simulink model "hexacopter"  (R2014a)
settings: Solver=ode45  StartTime=0.0  StopTime=100  MaxStep=0.5  RelTol=1e-3
undefined symbols (not defined in the file): g, Gt, K, M, m, MU0, obstacle, Qt, RangeFinderParam, Rt, SIGMA0, TP, vt
libraries: commnoisgen2 x2
settings Model: Creator=nirvana1289  LastModifiedBy=nirvana1289
settings DebuggingCC: UnderspecifiedInitializationDetection=Classic  StateNameClashWarn=warning

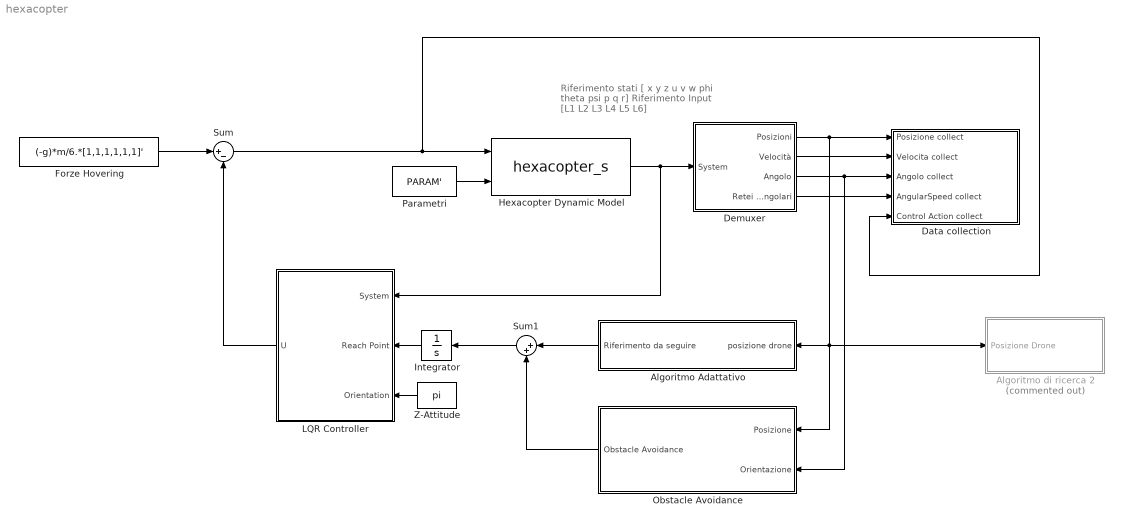
== system hexacopter ==
  note: Riferimento stati
      | [ x y z u v w phi theta psi p q r]
      | Riferimento Input
      | [L1 L2 L3 L4 L5 L6]
  Algoritmo Adattativo : Subsystem
  Algoritmo di ricerca 2 : Subsystem  Commented=on
  Data collection : Subsystem
  Demuxer : Subsystem
  Forze Hovering : Constant  Value=(-g)*m/6.*[1,1,1,1,1,1]'
  Hexacopter Dynamic Model : S-Function  InitFcn=try, set_param(gcb,'FunctionName','hexacopter_s'), end  FunctionName=hexacopter_s  SFunctionModules=hexacopter_s_wrapper  EnableBusSupport=off  mask(S-Function Builder){}
      mask help: Simulink:masks:SFunctionBuilder_MD
      mask init:
      | val = [[.9  0.75 0.75 1 1 .9 .9 1]',[1 1 0.75 0.75 .9 .9 1 .9]'];try , sys = get_param(gcb,'SfunBuilderFcnName');if isempty(sys), sys = get_param(gcb,'FunctionName'); end,catch, sys = get_param(gcb,'FunctionName'); end
      settings: CopyFcn=set_param(gcbh,'LinkStatus','none')  PreSaveFcn=try, set_param(gcb,'FunctionName','hexacopter_s'), end  OpenFcn=sfunctionwizard(gcbh)
      mask Display:
      | plot(val(:,1),val(:,2))
      | disp(sys)
      | port_label('input',1,'u')
      | port_label('input',2,'p')
      | port_label('output',1,'y')
  Integrator : Integrator  InitialCondition=RP'
  LQR Controller : Subsystem
  Obstacle Avoidance : Subsystem
  Parametri : Constant  Value=PARAM'
  Sum : Sum  Inputs=|+-
  Sum1 : Sum  Inputs=|++
  Z-Attitude : Constant  Value=pi
  wires:
  Sum/1 -> Hexacopter Dynamic Model/1, Data collection/5(Control Action collect)
  Forze Hovering/1 -> Sum/1
  Demuxer/3(Angolo) -> Obstacle Avoidance/2(Orientazione), Data collection/3(Angolo collect)
  Demuxer/4(Retei angolari) -> Data collection/4(AngularSpeed collect)
  Demuxer/2(Velocità) -> Data collection/2(Velocita collect)
  Demuxer/1(Posizioni) -> Obstacle Avoidance/1(Posizione), Algoritmo Adattativo/1(posizione drone), Algoritmo di ricerca 2/1(Posizione Drone), Data collection/1(Posizione collect)
  Parametri/1 -> Hexacopter Dynamic Model/2
  LQR Controller/1(U) -> Sum/2
  Z-Attitude/1 -> LQR Controller/3(Orientation)
  Hexacopter Dynamic Model/1 -> LQR Controller/1(System), Demuxer/1(System)
  Integrator/1 -> LQR Controller/2(Reach Point)
  Algoritmo Adattativo/1(Riferimento da seguire) -> Sum1/1
  Obstacle Avoidance/1(Obstacle Avoidance) -> Sum1/2
  Sum1/1 -> Integrator/1

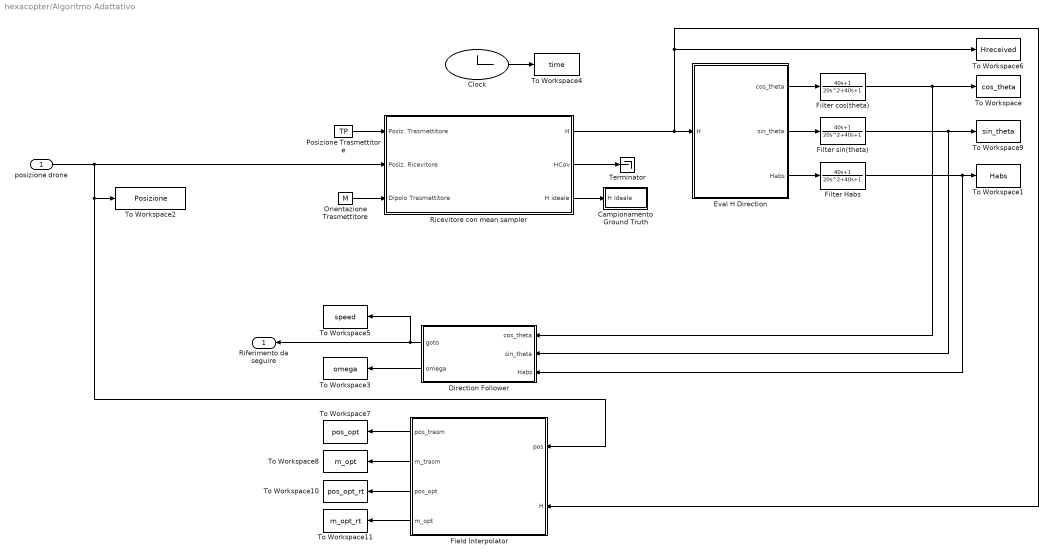
== system hexacopter/Algoritmo Adattativo ==
  posizione drone : Inport
  Campionamento Ground Truth : Subsystem
  Clock : Clock
  Direction Follower : MATLAB Function  TreatAsAtomicUnit=on
  Eval H Direction : MATLAB Function  TreatAsAtomicUnit=on
  Field Interpolator : MATLAB Function  TreatAsAtomicUnit=on
  Filter Habs : TransferFcn  Numerator=[40 1]  Denominator=[20,40,1]
  Filter cos(theta) : TransferFcn  Numerator=[40 1]  Denominator=[20,40,1]
  Filter sin(theta) : TransferFcn  Numerator=[40 1]  Denominator=[20,40,1]
  Orientazione Trasmettitore : Constant  Value=M
  Posizione Trasmettitore : Constant  Value=TP
  Ricevitore con mean sampler : Subsystem  TreatAsAtomicUnit=on
  Terminator : Terminator
  To Workspace : ToWorkspace  VariableName=cos_theta  SampleTime=-1
  To Workspace1 : ToWorkspace  VariableName=Habs  SampleTime=-1
  To Workspace10 : ToWorkspace  VariableName=pos_opt_rt  SampleTime=-1
  To Workspace11 : ToWorkspace  VariableName=m_opt_rt  SampleTime=-1
  To Workspace2 : ToWorkspace  VariableName=Posizione  SampleTime=-1
  To Workspace3 : ToWorkspace  VariableName=omega  SampleTime=-1
  To Workspace4 : ToWorkspace  VariableName=time  SampleTime=-1
  To Workspace5 : ToWorkspace  VariableName=speed  SampleTime=-1
  To Workspace6 : ToWorkspace  VariableName=Hreceived  SampleTime=-1
  To Workspace7 : ToWorkspace  VariableName=pos_opt  SampleTime=-1
  To Workspace8 : ToWorkspace  VariableName=m_opt  SampleTime=-1
  To Workspace9 : ToWorkspace  VariableName=sin_theta  SampleTime=-1
  Riferimento da seguire : Outport
  wires:
  Direction Follower/1(goto) -> Riferimento da seguire/1, To Workspace5/1
  Posizione Trasmettitore/1 -> Ricevitore con mean sampler/1(Posiz. Trasmettitore)
  Orientazione Trasmettitore/1 -> Ricevitore con mean sampler/3(Dipolo Trasmettitore)
  Eval H Direction/1(cos_theta) -> Filter cos(theta)/1
  posizione drone/1 -> Ricevitore con mean sampler/2(Posiz. Ricevitore), To Workspace2/1, Field Interpolator/1(pos)
  Ricevitore con mean sampler/2(HCov) -> Terminator/1
  Eval H Direction/3(Habs) -> Filter Habs/1
  Direction Follower/2(omega) -> To Workspace3/1
  Clock/1 -> To Workspace4/1
  Ricevitore con mean sampler/3(H ideale) -> Campionamento Ground Truth/1(H Ideale)
  Ricevitore con mean sampler/1(H) -> Field Interpolator/2(H), To Workspace6/1, Eval H Direction/1(H)
  Field Interpolator/1(pos_trasm) -> To Workspace7/1
  Field Interpolator/2(m_trasm) -> To Workspace8/1
  Eval H Direction/2(sin_theta) -> Filter sin(theta)/1
  Filter sin(theta)/1 -> Direction Follower/2(sin_theta), To Workspace9/1
  Filter Habs/1 -> Direction Follower/3(Habs), To Workspace1/1
  Filter cos(theta)/1 -> Direction Follower/1(cos_theta), To Workspace/1
  Field Interpolator/3(pos_opt) -> To Workspace10/1
  Field Interpolator/4(m_opt) -> To Workspace11/1

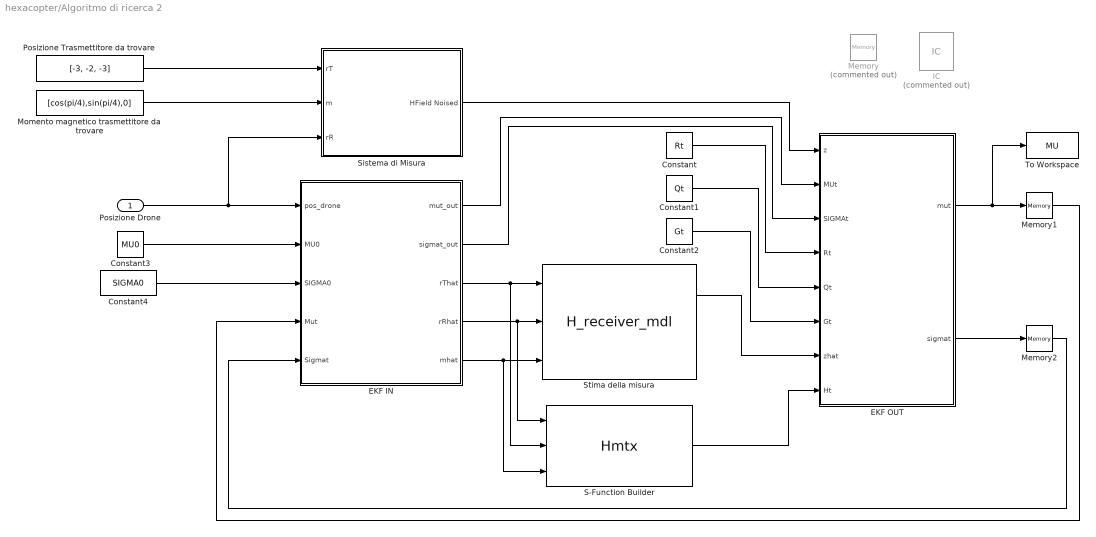
== system hexacopter/Algoritmo di ricerca 2 ==
  Posizione Drone : Inport
  Constant : Constant  Value=Rt
  Constant1 : Constant  Value=Qt
  Constant2 : Constant  Value=Gt
  Constant3 : Constant  Value=MU0
  Constant4 : Constant  Value=SIGMA0
  EKF IN : MATLAB Function  TreatAsAtomicUnit=on
  EKF OUT : MATLAB Function  TreatAsAtomicUnit=on
  IC : InitialCondition  Commented=on
  Memory : Memory  Commented=on
  Memory1 : Memory  X0=zeros(9,1)
  Memory2 : Memory  X0=ones(9,9)
  Momento magnetico trasmettitore da trovare : Constant  Value=[cos(pi/4),sin(pi/4),0]
  Posizione Trasmettitore da trovare : Constant  Value=[-3, -2, -3]
  S-Function Builder : S-Function  InitFcn=try, set_param(gcb,'FunctionName','Hmtx'), end  FunctionName=Hmtx  SFunctionModules=Hmtx_wrapper  EnableBusSupport=off  mask(S-Function Builder){}
      mask help: Simulink:masks:SFunctionBuilder_MD
      mask init: same as hexacopter/Hexacopter Dynamic Model
      settings: CopyFcn=set_param(gcbh,'LinkStatus','none')  PreSaveFcn=try, set_param(gcb,'FunctionName','Hmtx'), end  OpenFcn=sfunctionwizard(gcbh)
      mask Display: plot(val(:,1),val(:,2)),disp(sys), port_label('input',1,'rR'), port_label('input',2,'rT'), port_label('input',3,'m'), port_label('output',1,'HMtx')
  Sistema di Misura : Subsystem
  Stima della misura : S-Function  FunctionName=H_receiver_mdl  EnableBusSupport=off
  To Workspace : ToWorkspace  VariableName=MU  SampleTime=-1
  wires:
  Posizione Drone/1 -> EKF IN/1(pos_drone), Sistema di Misura/3(rR)
  Constant3/1 -> EKF IN/2(MU0)
  Constant4/1 -> EKF IN/3(SIGMA0)
  Posizione Trasmettitore da trovare/1 -> Sistema di Misura/1(rT)
  Momento magnetico trasmettitore da trovare/1 -> Sistema di Misura/2(m)
  EKF IN/5(mhat) -> S-Function Builder/3, Stima della misura/3
  EKF IN/3(rThat) -> S-Function Builder/2, Stima della misura/1
  EKF IN/4(rRhat) -> S-Function Builder/1, Stima della misura/2
  Sistema di Misura/1(HField Noised) -> EKF OUT/1(z)
  EKF IN/1(mut_out) -> EKF OUT/2(MUt)
  EKF IN/2(sigmat_out) -> EKF OUT/3(SIGMAt)
  Constant/1 -> EKF OUT/4(Rt)
  Constant1/1 -> EKF OUT/5(Qt)
  Constant2/1 -> EKF OUT/6(Gt)
  Stima della misura/1 -> EKF OUT/7(zhat)
  S-Function Builder/1 -> EKF OUT/8(Ht)
  EKF OUT/1(mut) -> To Workspace/1, Memory1/1
  EKF OUT/2(sigmat) -> Memory2/1
  Memory2/1 -> EKF IN/5(Sigmat)
  Memory1/1 -> EKF IN/4(Mut)

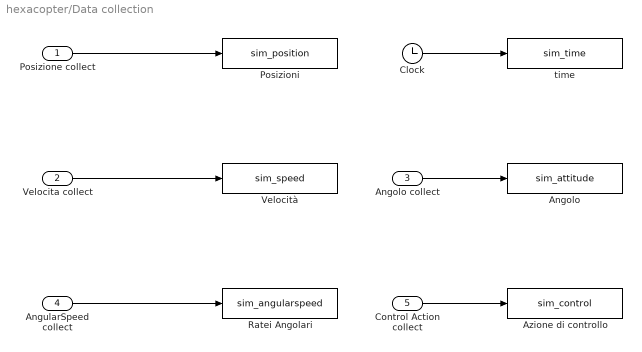
== system hexacopter/Data collection ==
  Posizione collect : Inport
  Velocita collect : Inport  Port=2
  Angolo collect : Inport  Port=3
  AngularSpeed collect : Inport  Port=4
  Control Action collect : Inport  Port=5
  Angolo : ToWorkspace  VariableName=sim_attitude  SampleTime=-1
  Azione di controllo : ToWorkspace  VariableName=sim_control  SampleTime=-1
  Clock : Clock
  "Posizioni " : ToWorkspace  VariableName=sim_position  SampleTime=-1
  Ratei Angolari : ToWorkspace  VariableName=sim_angularspeed  SampleTime=-1
  Velocità : ToWorkspace  VariableName=sim_speed  SampleTime=-1
  time : ToWorkspace  VariableName=sim_time  SampleTime=-1
  wires:
  Angolo collect/1 -> Angolo/1
  Posizione collect/1 -> "Posizioni "/1
  AngularSpeed collect/1 -> Ratei Angolari/1
  Velocita collect/1 -> Velocità/1
  Clock/1 -> time/1
  Control Action collect/1 -> Azione di controllo/1

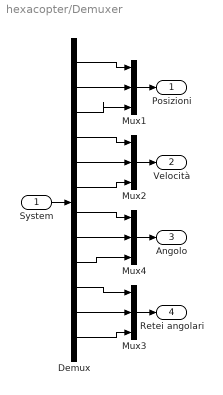
== system hexacopter/Demuxer ==
  System : Inport
  Demux : Demux  Outputs=12
  Mux{1..4} (4 alike) : Mux  Inputs=3
  Posizioni : Outport
  Velocità : Outport  Port=2
  Angolo : Outport  Port=3
  Retei angolari : Outport  Port=4
  wires:
  System/1 -> Demux/1
  Demux/2 -> Mux1/2
  Demux/12 -> Mux3/3
  Mux1/1 -> Posizioni/1
  Demux/7 -> Mux4/1
  Mux4/1 -> Angolo/1
  Demux/11 -> Mux3/2
  Demux/1 -> Mux1/1
  Demux/3 -> Mux1/3
  Mux3/1 -> Retei angolari/1
  Demux/10 -> Mux3/1
  Demux/5 -> Mux2/2
  Demux/9 -> Mux4/3
  Mux2/1 -> Velocità/1
  Demux/8 -> Mux4/2
  Demux/6 -> Mux2/3
  Demux/4 -> Mux2/1

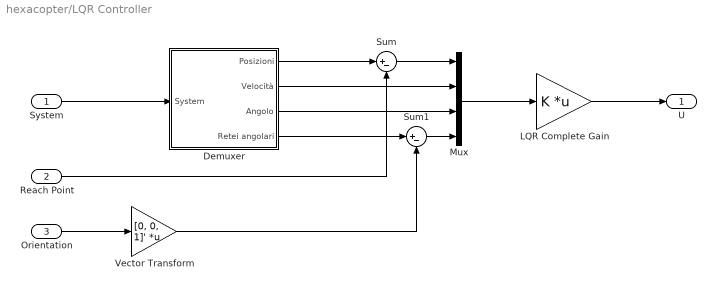
== system hexacopter/LQR Controller ==
  System : Inport
  Reach Point : Inport  Port=2
  Orientation : Inport  Port=3
  Demuxer : Subsystem
  LQR Complete Gain : Gain  Gain=K  Multiplication=Matrix(K*u)
  Mux : Mux
  Sum : Sum  Inputs=|+-
  Sum1 : Sum  Inputs=|+-
  Vector Transform : Gain  Gain=[0, 0, 1]'  Multiplication=Matrix(K*u)
  U : Outport
  wires:
  Mux/1 -> LQR Complete Gain/1
  Reach Point/1 -> Sum/2
  Orientation/1 -> Vector Transform/1
  Vector Transform/1 -> Sum1/2
  Demuxer/1(Posizioni) -> Sum/1
  Demuxer/2(Velocità) -> Mux/2
  Demuxer/3(Angolo) -> Mux/3
  Demuxer/4(Retei angolari) -> Sum1/1
  Sum1/1 -> Mux/4
  Sum/1 -> Mux/1
  System/1 -> Demuxer/1(System)
  LQR Complete Gain/1 -> U/1

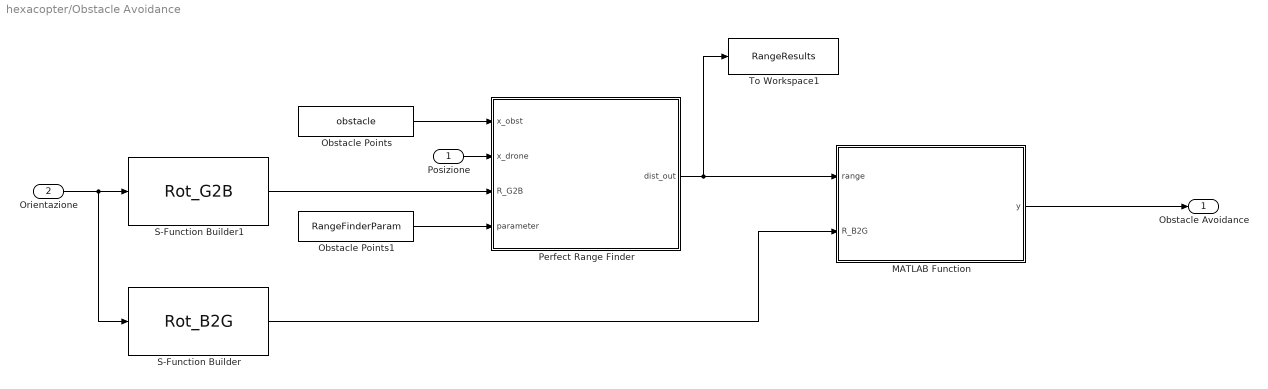
== system hexacopter/Obstacle Avoidance ==
  Posizione : Inport
  Orientazione : Inport  Port=2
  MATLAB Function : MATLAB Function  TreatAsAtomicUnit=on
  Obstacle Points : Constant  Value=obstacle
  Obstacle Points1 : Constant  Value=RangeFinderParam
  Perfect Range Finder : MATLAB Function  TreatAsAtomicUnit=on
  S-Function Builder : S-Function  InitFcn=try, set_param(gcb,'FunctionName','Rot_G2B'), end  FunctionName=Rot_B2G  SFunctionModules=Rot_B2G_wrapper  EnableBusSupport=off  mask(S-Function Builder){}
      mask help: Simulink:masks:SFunctionBuilder_MD
      mask init: same as hexacopter/Hexacopter Dynamic Model
      settings: CopyFcn=set_param(gcbh,'LinkStatus','none')  PreSaveFcn=try, set_param(gcb,'FunctionName','Rot_B2G'), end  OpenFcn=sfunctionwizard(gcbh)
      mask Display: plot(val(:,1),val(:,2)),disp(sys), port_label('input',1,'angles'), port_label('output',1,'rot')
  S-Function Builder1 : S-Function  InitFcn=try, set_param(gcb,'FunctionName','Rot_G2B'), end  FunctionName=Rot_G2B  SFunctionModules=Rot_G2B_wrapper  EnableBusSupport=off  mask(S-Function Builder){}
      mask help: Simulink:masks:SFunctionBuilder_MD
      mask init: same as hexacopter/Hexacopter Dynamic Model
      settings: CopyFcn=set_param(gcbh,'LinkStatus','none')  PreSaveFcn=try, set_param(gcb,'FunctionName','Rot_G2B'), end  OpenFcn=sfunctionwizard(gcbh)
      mask Display:
      | plot(val(:,1),val(:,2))
      | disp(sys)
      | port_label('input',1,'angles')
      | port_label('output',1,'rot')
  To Workspace1 : ToWorkspace  VariableName=RangeResults  SampleTime=-1
  Obstacle Avoidance : Outport
  wires:
  Orientazione/1 -> S-Function Builder/1, S-Function Builder1/1
  Obstacle Points1/1 -> Perfect Range Finder/4(parameter)
  Perfect Range Finder/1(dist_out) -> MATLAB Function/1(range), To Workspace1/1
  S-Function Builder1/1 -> Perfect Range Finder/3(R_G2B)
  Posizione/1 -> Perfect Range Finder/2(x_drone)
  Obstacle Points/1 -> Perfect Range Finder/1(x_obst)
  S-Function Builder/1 -> MATLAB Function/2(R_B2G)
  MATLAB Function/1(y) -> Obstacle Avoidance/1

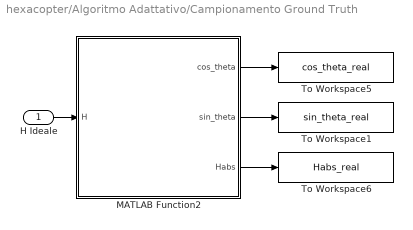
== system hexacopter/Algoritmo Adattativo/Campionamento Ground Truth ==
  H Ideale : Inport
  MATLAB Function2 : MATLAB Function  TreatAsAtomicUnit=on
  To Workspace1 : ToWorkspace  VariableName=sin_theta_real  SampleTime=-1
  To Workspace5 : ToWorkspace  VariableName=cos_theta_real  SampleTime=-1
  To Workspace6 : ToWorkspace  VariableName=Habs_real  SampleTime=-1
  wires:
  MATLAB Function2/3(Habs) -> To Workspace6/1
  H Ideale/1 -> MATLAB Function2/1(H)
  MATLAB Function2/1(cos_theta) -> To Workspace5/1
  MATLAB Function2/2(sin_theta) -> To Workspace1/1

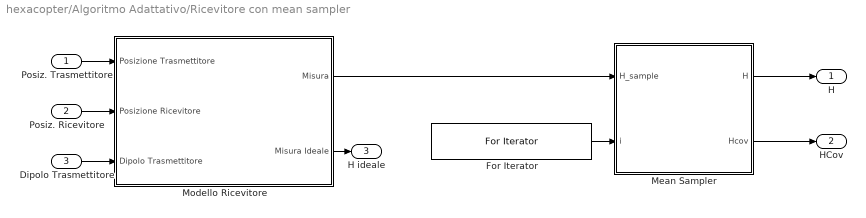
== system hexacopter/Algoritmo Adattativo/Ricevitore con mean sampler ==
  Posiz. Trasmettitore : Inport
  Posiz. Ricevitore : Inport  Port=2
  Dipolo Trasmettitore : Inport  Port=3
  For Iterator : ForIterator  IterationLimit=50
  Mean Sampler : MATLAB Function  TreatAsAtomicUnit=on
  Modello Ricevitore : Subsystem
  H : Outport
  HCov : Outport  Port=2
  H ideale : Outport  Port=3
  wires:
  Dipolo Trasmettitore/1 -> Modello Ricevitore/3(Dipolo Trasmettitore)
  Modello Ricevitore/1(Misura) -> Mean Sampler/1(H_sample)
  Mean Sampler/1(H) -> H/1
  Posiz. Trasmettitore/1 -> Modello Ricevitore/1(Posizione Trasmettitore)
  Mean Sampler/2(Hcov) -> HCov/1
  Posiz. Ricevitore/1 -> Modello Ricevitore/2(Posizione Ricevitore)
  For Iterator/1 -> Mean Sampler/2(i)
  Modello Ricevitore/2(Misura Ideale) -> H ideale/1

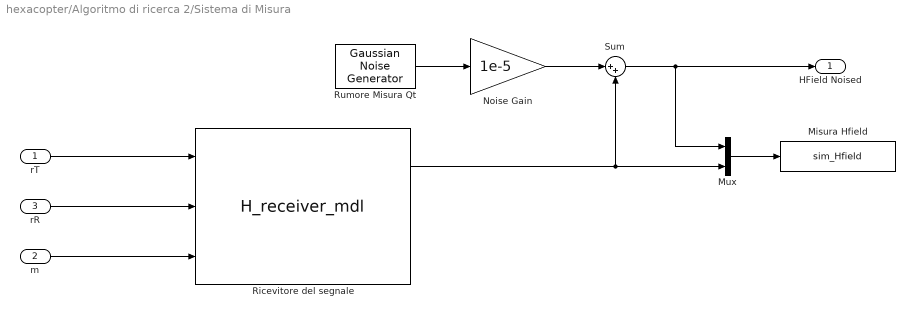
== system hexacopter/Algoritmo di ricerca 2/Sistema di Misura ==
  rT : Inport
  m : Inport  Port=2
  rR : Inport  Port=3
  Misura Hfield : ToWorkspace  VariableName=sim_Hfield  SampleTime=-1
  Mux : Mux  Inputs=2
  Noise Gain : Gain  Gain=1e-5
  Ricevitore del segnale : S-Function  InitFcn=try, set_param(gcb,'FunctionName','H_receiver_mdl'), end  FunctionName=H_receiver_mdl  SFunctionModules=H_receiver_mdl_wrapper  EnableBusSupport=off  mask(S-Function Builder){}
      mask help: Simulink:masks:SFunctionBuilder_MD
      mask init: same as hexacopter/Hexacopter Dynamic Model
      settings: CopyFcn=set_param(gcbh,'LinkStatus','none')  PreSaveFcn=try, set_param(gcb,'FunctionName','H_receiver_mdl'), end  OpenFcn=sfunctionwizard(gcbh)
      mask Display: plot(val(:,1),val(:,2)),disp(sys), port_label('input',1,'rT'), port_label('input',2,'rR'), port_label('input',3,'m'), port_label('output',1,'HField'), port_label('output',2,'Hstrenght')
  Rumore Misura Qt : commnoisgen2/Gaussian Noise Generator  m=vt  d=Qt  s=41  Ts=1  frameBased=off  sampPerFrame=1  orient=off  outDataType=double
  Sum : Sum  Inputs=|++
  HField Noised : Outport
  wires:
  Mux/1 -> Misura Hfield/1
  Ricevitore del segnale/1 -> Mux/2, Sum/2
  Sum/1 -> HField Noised/1, Mux/1
  Rumore Misura Qt/1 -> Noise Gain/1
  Noise Gain/1 -> Sum/1
  rT/1 -> Ricevitore del segnale/1
  rR/1 -> Ricevitore del segnale/2
  m/1 -> Ricevitore del segnale/3

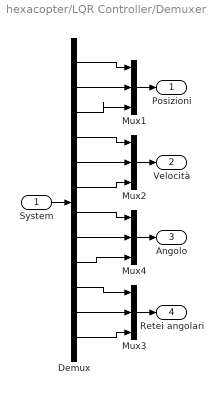
== system hexacopter/LQR Controller/Demuxer ==
  System : Inport
  Demux : Demux  Outputs=12
  Mux{1..4} (4 alike) : Mux  Inputs=3
  Posizioni : Outport
  Velocità : Outport  Port=2
  Angolo : Outport  Port=3
  Retei angolari : Outport  Port=4
  wires:
  System/1 -> Demux/1
  Demux/2 -> Mux1/2
  Demux/12 -> Mux3/3
  Mux1/1 -> Posizioni/1
  Demux/7 -> Mux4/1
  Mux4/1 -> Angolo/1
  Demux/11 -> Mux3/2
  Demux/1 -> Mux1/1
  Demux/3 -> Mux1/3
  Mux3/1 -> Retei angolari/1
  Demux/10 -> Mux3/1
  Demux/5 -> Mux2/2
  Demux/9 -> Mux4/3
  Mux2/1 -> Velocità/1
  Demux/8 -> Mux4/2
  Demux/6 -> Mux2/3
  Demux/4 -> Mux2/1

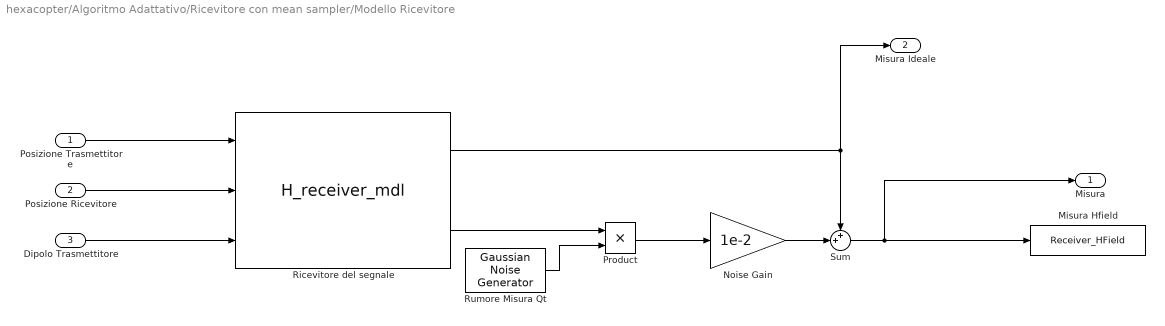
== system hexacopter/Algoritmo Adattativo/Ricevitore con mean sampler/Modello Ricevitore ==
  Posizione Trasmettitore : Inport
  Posizione Ricevitore : Inport  Port=2
  Dipolo Trasmettitore : Inport  Port=3
  Misura Hfield : ToWorkspace  VariableName=Receiver_HField  SampleTime=-1
  Noise Gain : Gain  Gain=1e-2
  Product : Product
  Ricevitore del segnale : S-Function  InitFcn=try, set_param(gcb,'FunctionName','H_receiver_mdl'), end  FunctionName=H_receiver_mdl  SFunctionModules=H_receiver_mdl_wrapper  EnableBusSupport=off  mask(S-Function Builder){}
      mask help: Simulink:masks:SFunctionBuilder_MD
      mask init: same as hexacopter/Hexacopter Dynamic Model
      settings: CopyFcn=set_param(gcbh,'LinkStatus','none')  PreSaveFcn=try, set_param(gcb,'FunctionName','H_receiver_mdl'), end  OpenFcn=sfunctionwizard(gcbh)
      mask Display:
      | plot(val(:,1),val(:,2))
      | disp(sys)
      | port_label('input',1,'rT')
      | port_label('input',2,'rR')
      | port_label('input',3,'m')
      | port_label('output',1,'HField')
      | port_label('output',2,'Hstrenght')
  Rumore Misura Qt : commnoisgen2/Gaussian Noise Generator  m=vt  d=Qt  s=41  Ts=-1  frameBased=off  sampPerFrame=1  orient=off  outDataType=double
  Sum : Sum  Inputs=++|
  Misura : Outport
  Misura Ideale : Outport  Port=2
  wires:
  Ricevitore del segnale/2 -> Product/1
  Rumore Misura Qt/1 -> Product/2
  Posizione Ricevitore/1 -> Ricevitore del segnale/2
  Dipolo Trasmettitore/1 -> Ricevitore del segnale/3
  Sum/1 -> Misura/1, Misura Hfield/1
  Ricevitore del segnale/1 -> Sum/1, Misura Ideale/1
  Noise Gain/1 -> Sum/2
  Posizione Trasmettitore/1 -> Ricevitore del segnale/1
  Product/1 -> Noise Gain/1

== matlab function hexacopter/Algoritmo di ricerca 2/EKF IN ==
  data: pos_drone input; mut_out output; sigmat_out output; rThat output; rRhat output; MU0 input; SIGMA0 input; mhat output; Mut input; Sigmat input
function [mut_out,sigmat_out, rThat, rRhat, mhat] = ekf_wrapper_in(pos_drone ,MU0, SIGMA0, Mut, Sigmat)
%#codegen
    persistent MUt;
    if isempty(MUt);
        MUt = MU0;
    else
        MUt = Mut;
        MUt(1:3) = pos_drone;
    end
    
    persistent SIGMAt;
    if isempty(SIGMAt)
        SIGMAt = SIGMA0;
    else
        SIGMAt = Sigmat;
    end
    
    mut_out = MUt+zeros(9,1);
    sigmat_out = SIGMAt+zeros(9,9);
    rRhat = MUt(1:3);
    rThat = MUt(4:6);
    mhat  = MUt(7:9);

== matlab function hexacopter/Algoritmo Adattativo/Eval H Direction ==
  data: H input; cos_theta output; sin_theta output; Habs output
function [cos_theta,sin_theta,Habs] = HDirection(H)
%#codegen
    
    persistent theta_memory;
    if isempty(theta_memory)
        theta_memory = atan2(H(2),H(1));
    end

    
    theta = atan2(H(2),H(1));

    cos_theta=cos(theta);
    sin_theta=sin(theta);  
       
    
    Habs = sqrt(sum(H.^2));

== matlab function hexacopter/Algoritmo di ricerca 2/EKF OUT ==
  data: z input; MUt input; SIGMAt input; Rt input; mut output; Qt input; Gt input; zhat input; Ht input; sigmat output
function [mut,sigmat] = ekf_wrapper_out(z,MUt,SIGMAt,Rt,Qt,Gt,zhat,Ht)
%#codegen
    
    [mut,sigmat,~,~,~] = ekf(MUt,SIGMAt,Ht,Gt,z,zhat,Rt,Qt);

== matlab function hexacopter/Algoritmo Adattativo/Direction Follower ==
  data: cos_theta input; sin_theta input; goto output; Habs input; omega output
function [goto,omega] = direction_finder(cos_theta,sin_theta,Habs)
    
    B = 0.3;
    A = 0.05;
    alpha = 0.2;
    beta = 0.35;

    persistent psi;
    if isempty(psi)
        psi = atan2(sin_theta,cos_theta);
    end
    persistent Hprev;
    if isempty(Hprev)
        Hprev = 0;
    end
    persistent speed
    if isempty(speed)
        speed = 1;
    end
    
    if ((Habs/Hprev) - 1 > beta)
        psi = (1-alpha)*psi + alpha*B;
    elseif ((Habs/Hprev) - 1 < -beta);
        psi = (1-alpha)*psi - alpha*B;
    end
    speed = (1-beta)*speed + beta*A*log(Habs+1e-15);
    
    cos_omega = (1-alpha)*cos_theta+alpha*cos(psi);
    sin_omega = (1-alpha)*sin_theta+alpha*sin(psi);
    
    omega = atan2(sin_omega,cos_omega);
    goto = [ speed*cos_omega, speed*sin_omega,0 ]';

== matlab function hexacopter/Algoritmo Adattativo/Campionamento Ground Truth/MATLAB Function2 ==
  data: H input; cos_theta output; sin_theta output; Habs output
function [cos_theta,sin_theta,Habs] = HDirection(H)
%#codegen

    theta = atan2(H(2),H(1));
    Habs = sqrt(sum(H.^2));
    cos_theta = cos(theta);
    sin_theta = sin(theta);

== matlab function hexacopter/Algoritmo Adattativo/Field Interpolator ==
  data: pos input; pos_trasm output; H input; m_trasm output; pos_opt output; m_opt output
function [pos_trasm, m_trasm, pos_opt, m_opt] = position_appoximation2(pos,H)
%#codegen
    coder.extrinsic('optimizer2');
    MEMORY = 4;
    
    % Apprendimento dell'algoritmo
    alpha = 0.3;

    optimized_vector = zeros(6,1);
    persistent counter
    persistent Hfield_memory;
    persistent Rposition_memory;
    persistent RT;
    persistent M;
       
    if isempty(counter)
        counter = 0;
    end
    % Memory allocation
    if isempty(Hfield_memory)
        Hfield_memory = zeros(MEMORY,3);
    end
    if isempty(Rposition_memory)
        Rposition_memory = zeros(MEMORY,3);
    end

    % Results allocation
    if isempty(RT)
        RT = [0, 0, 0];
    end
    if isempty(M)
        M = [0,0,0];
    end 

    counter = counter + 1;
    Hfield_memory(counter,:) = H;
    Rposition_memory(counter,:) = pos;
    if counter == MEMORY
        counter = 0;
        optimized = feval('optimizer2',Rposition_memory', Hfield_memory', [RT, M]');
        optimized_vector = optimized;
        RT = (1-alpha)*RT + alpha*optimized_vector(1:3)';
        M = (1-alpha)*M + alpha*optimized_vector(1:3)';
    end
    
    pos_trasm = RT;
    m_trasm = M;
    pos_opt = optimized_vector(1:3);
    m_opt = optimized_vector(4:6);

== matlab function hexacopter/Algoritmo Adattativo/Ricevitore con mean sampler/Mean Sampler ==
  data: H_sample input; H output; i input; Hcov output
function [H, Hcov] = media(H_sample, i)
%#codegen
    n = 50;

    persistent HVECTOR;
    persistent HMEAN;
    persistent HCOVARIANCE;
    if isempty(HVECTOR);
        HVECTOR = zeros(3,n);
    end
    if isempty(HMEAN)
        HMEAN = zeros(3,1);
    end
    if isempty(HCOVARIANCE)
        HCOVARIANCE = zeros(3,3);
    end
    
    h_tmp = zeros(3,1);
    cov_tmp = zeros(3,n);
    
    if i == n
        % Eval mean
        HMEAN = 1/n * sum(HVECTOR,2);
        % Eval covariance
        for j = 1:n
            cov_tmp(:,j) = HVECTOR(:,j) - HMEAN(:);
            HCOVARIANCE = HCOVARIANCE + cov_tmp(:,j)'*cov_tmp(:,1);
        end
        HCOVARIANCE = 1/n*HCOVARIANCE;
    else
        HVECTOR(:,i) = H_sample;
    end
    
    H = HMEAN+zeros(3,1);
    Hcov = HCOVARIANCE+zeros(3,3);

== matlab function hexacopter/Obstacle Avoidance/Perfect Range Finder ==
  data: x_obst input; dist_out output; x_drone input; R_G2B input; parameter input
function dist_out = rangeFinder(x_obst, x_drone, R_G2B, parameter)
    dist_out = zeros(6,1);
    d = zeros(size(x_obst));
    dist = zeros(6,size(x_obst,2));
    h = parameter(1);
    rho = parameter(2);
    
    for i = 1:size(x_obst,2)
       d(:,i) = R_G2B*(x_obst(:,i) - x_drone);
       didi = d(:,i)' * d(:,i);
       for j = 1:6 
          dist(j,i) = cos((j-1)*pi/3)*d(1,i) - sin((j-1)*pi/3)*d(2,i);
          if and(dist(j,i) >= 0, dist(j,i) <= h)
              if didi - dist(j,i)^2 - ((h-dist(j,i))*rho/h)^2 >= 0
                  dist(j,i) = inf;
              end
          else 
               dist(j,i) = inf;
          end
       end
    end
    for i = 1:6
        dist_out(i) = min(dist(i,:));
    end
end

== matlab function hexacopter/Obstacle Avoidance/MATLAB Function ==
  data: range input; y output; R_B2G input
function y = ObsAvoidSpeed(range, R_B2G)
%#codegen
    y = zeros(3,1);
    for i=1:6
        y = y - 1/range(i).*[ cos((i-1)*pi/3); -sin((i-1)*pi/3); 0 ];
    end
    y = R_B2G*y;
